simulink model "Practica3_MovimientoTraslacional_Sim"  (R2022b)
settings: Solver=ode45  StartTime=0.0  StopTime=10.0  MaxStep=0.001  RelTol=1e-3
values from neighbouring files (symbols this model uses):
  b1 = 1000    [MovimientoTraslacional.m]    (also in Practica3_MovimientoTraslacional_MSim.m)
  f = 0    [MovimientoTraslacional.m]    (also in Practica3_MovimientoTraslacional_MSim.m)
  k1 = 16182    [MovimientoTraslacional.m]    (also in Practica3_MovimientoTraslacional_MSim.m)
  k2 = 19000    [MovimientoTraslacional.m]    (also in Practica3_MovimientoTraslacional_MSim.m)
  m1 = 290    [MovimientoTraslacional.m]    (also in Practica3_MovimientoTraslacional_MSim.m)
  m2 = 59    [MovimientoTraslacional.m]    (also in Practica3_MovimientoTraslacional_MSim.m)
settings Model: Creator=mluser  LastModifiedBy=mluser

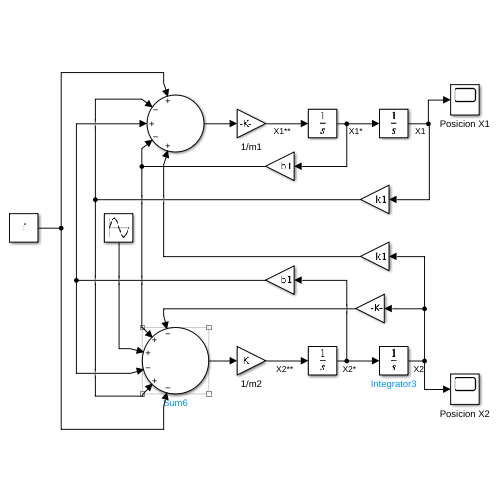
[thumbnail: Simulink's stored preview of the top-level diagram]
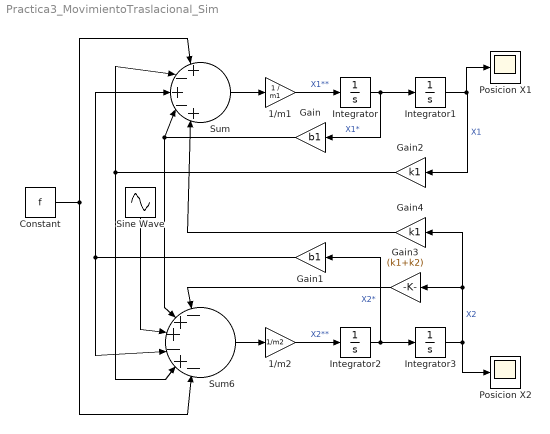
== system Practica3_MovimientoTraslacional_Sim ==
  1/m1 : Gain  Gain=1 / m1
  1/m2 : Gain  Gain=1/m2
  Constant : Constant  Value=f
  Gain : Gain  Gain=b1
  Gain1 : Gain  Gain=b1
  Gain2 : Gain  Gain=k1
  Gain3 : Gain  Gain=(k1+k2)
  Gain4 : Gain  Gain=k1
  Integrator{,1..3} (4 alike) : Integrator
  Posicion X1 : Scope
  Posicion X2 : Scope
  Sine Wave : Sin  Amplitude=0.05*k2  Frequency=0.5*pi  SampleTime=0
  Sum : Sum  Inputs=|+|-|+|-|+|
  Sum6 : Sum  Inputs=|-|+|+|-|+|-|
  wires:
  Sum/1 -> 1/m1/1
  1/m2/1 -> Integrator2/1  "X2**"
  Integrator2/1 -> Integrator3/1, Gain1/1  "X2*"
  Sum6/1 -> 1/m2/1
  Integrator/1 -> Integrator1/1, Gain/1  "X1*"
  Integrator1/1 -> Posicion X1/1, Gain2/1  "X1"
  1/m1/1 -> Integrator/1  "X1**"
  Integrator3/1 -> Gain4/1, Gain3/1, Posicion X2/1  "X2"
  Constant/1 -> Sum/1, Sum6/6
  Gain/1 -> Sum/4, Sum6/2
  Gain1/1 -> Sum6/4, Sum/3
  Gain2/1 -> Sum/2, Sum6/5
  Sine Wave/1 -> Sum6/3
  Gain4/1 -> Sum/5
  Gain3/1 -> Sum6/1
